simulink model "WindTunnel"  (R2016b)
settings: Solver=VariableStepAuto  StartTime=0.0  StopTime=20  MaxStep=0.01  RelTol=1e-3
undefined symbols (not defined in the file or in its folder): P, Scale
libraries: simulink x1
settings Model: Creator=CFRPG  LastModifiedBy=CFRPG

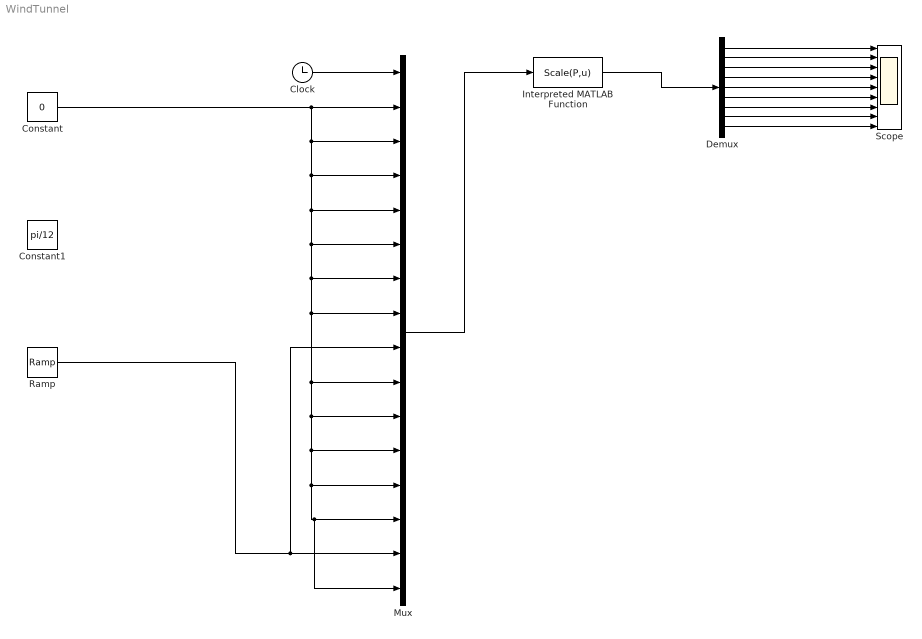
== system WindTunnel ==
  Clock : Clock
  Constant : Constant  Value=0
  Constant1 : Constant  Value=pi/12
  Demux : Demux  Outputs=9
  Interpreted MATLAB Function : MATLABFcn  MATLABFcn=Scale(P,u)
  Mux : Mux  Inputs=16
  Ramp : simulink/Sources/Ramp  slope=pi/10  start=0  X0=0
  Scope : Scope  NumInputPorts=9
  wires:
  Mux/1 -> Interpreted MATLAB Function/1
  Constant/1 -> Mux/7, Mux/10, Mux/11, Mux/12, Mux/13, Mux/16, Mux/14, Mux/8, Mux/6, Mux/5, Mux/4, Mux/3, Mux/2
  Clock/1 -> Mux/1
  Interpreted MATLAB Function/1 -> Demux/1
  Demux/1 -> Scope/1
  Demux/2 -> Scope/2
  Demux/3 -> Scope/3
  Demux/4 -> Scope/4
  Ramp/1 -> Mux/9, Mux/15
  Demux/5 -> Scope/5
  Demux/6 -> Scope/6
  Demux/7 -> Scope/7
  Demux/8 -> Scope/8
  Demux/9 -> Scope/9
